simulink model "Arrays3"  (Simulink 5.0)
settings: Solver=FixedStepDiscrete  StartTime=0.0  StopTime=10000.0  RelTol=1e-3
settings Model: Creator=scaife  LastModifiedBy=scaife  ExtModeAutoUpdateStatusClock=off

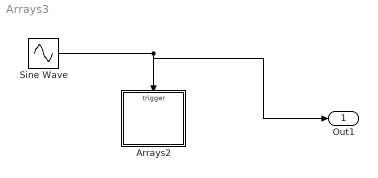
== system Arrays3 ==
  Arrays2 : Stateflow chart
  Sine Wave : Sin  SampleTime=0
  Out1 : Outport
  wires:
  Sine Wave/1 -> Arrays2/Trigger, Out1/1

== stateflow chart Arrays2 ==
  state A/
    en:x[1][1][1]++
    x[1][1][2]+=2
    x[1][2][1]+=3
    x[1][2][2]+=4
  state B/
    en:x[2][1][1]++
    x[2][1][2]+=2
    x[2][2][1]+=3
    x[2][2][2]+=4
  state C/
    en:x[3][1][1]++
    x[3][1][2]+=2
    x[3][2][1]+=3
    x[3][2][2]+=4
  (default) -> A
  A -> B : E
  B -> C : E
  C -> A : E
  data: x local int32 size=3 2 2 [0..100] =1
  events: E input RISING_EDGE_EVENT
